simulink model "FODTfiiting"  (R2019a)
settings: Solver=ode2  StartTime=0.0  StopTime=300  FixedStep=0.1  RelTol=1e-3
settings Model: Creator=HP  LastModifiedBy=swastik
settings DataIOCC: ReturnWorkspaceOutputs=off
settings DebuggingCC: ArithmeticOperatorsInVariantConditions=warning

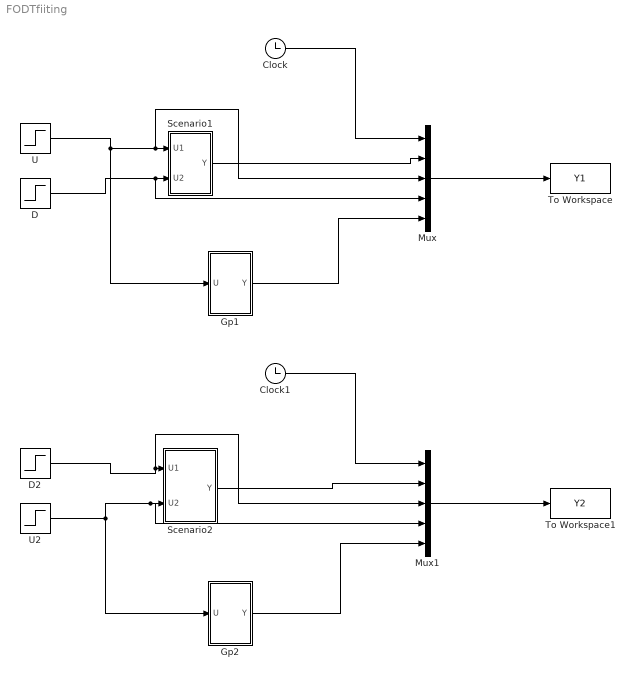
== system FODTfiiting ==
  Clock : Clock
  Clock1 : Clock
  D : Step  Time=0  After=0  SampleTime=0
  D2 : Step  Time=0  After=0  SampleTime=0
  Gp1 : Subsystem  mask{K=1.9886, T=17.4, D=14}
      mask prompts: K "Gain"; T "Lag Time"; D "Dead Time"
  Gp2 : Subsystem  mask{K2=0.9894, T2=26.1, D2=20.6}
      mask prompts: K2 "Gain"; T2 "Lag time"; D2 "Dead Time"
  Mux : Mux  Inputs=5
  Mux1 : Mux  Inputs=5
  Scenario1 : Subsystem
  Scenario2 : Subsystem
  To Workspace : ToWorkspace  VariableName=Y1  SampleTime=-1
  To Workspace1 : ToWorkspace  VariableName=Y2  SampleTime=-1
  U : Step  Time=0  SampleTime=0
  U2 : Step  Time=0  SampleTime=0
  wires:
  U/1 -> Gp1/1(U), Mux/3, Scenario1/1(U1)
  D/1 -> Mux/4, Scenario1/2(U2)
  Clock/1 -> Mux/1
  Scenario1/1(Y) -> Mux/2
  Mux/1 -> To Workspace/1
  Mux1/1 -> To Workspace1/1
  Scenario2/1(Y) -> Mux1/2
  D2/1 -> Mux1/3, Scenario2/1(U1)
  U2/1 -> Gp2/1(U), Mux1/4, Scenario2/2(U2)
  Clock1/1 -> Mux1/1
  Gp1/1(Y) -> Mux/5
  Gp2/1(Y) -> Mux1/5

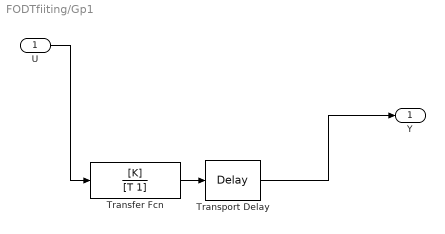
== system FODTfiiting/Gp1 ==
  U : Inport
  Transfer Fcn : TransferFcn  Numerator=[K]  Denominator=[T 1]
  Transport Delay : TransportDelay  DelayTime=D
  Y : Outport
  wires:
  Transfer Fcn/1 -> Transport Delay/1
  U/1 -> Transfer Fcn/1
  Transport Delay/1 -> Y/1

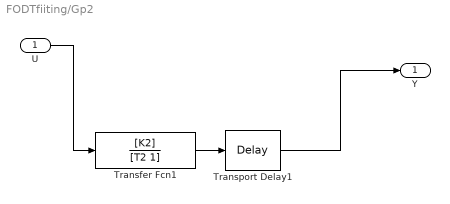
== system FODTfiiting/Gp2 ==
  U : Inport
  Transfer Fcn1 : TransferFcn  Numerator=[K2]  Denominator=[T2 1]
  Transport Delay1 : TransportDelay  DelayTime=D2
  Y : Outport
  wires:
  Transfer Fcn1/1 -> Transport Delay1/1
  Transport Delay1/1 -> Y/1
  U/1 -> Transfer Fcn1/1

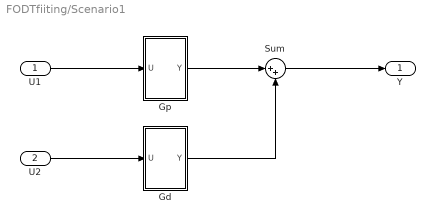
== system FODTfiiting/Scenario1 ==
  U1 : Inport
  U2 : Inport  Port=2
  Gd : Subsystem  mask{K1=0.45, K2=0.45, T1=0.3, T2=0.3, K=1/17e-4}
      mask prompts: K1 "Forward Gain"; K2 "Rev Gain"; T1 "Forward Time Constt"; T2 "Rev Time Constt"; K "Scaling Gain"
  Gp : Subsystem  mask{K1=0.45, K2=0.45, T1=0.2, T2=0.2, K=2.01/17e-4}
      mask prompts: K1 "Forward Gain"; K2 "Rev Gain"; T1 "Forward Time Constt"; T2 "Rev Time Constt"; K "Scaling Gain"
  Sum : Sum  Inputs=|++
  Y : Outport
  wires:
  Gd/1(Y) -> Sum/2
  Sum/1 -> Y/1
  Gp/1(Y) -> Sum/1
  U1/1 -> Gp/1(U)
  U2/1 -> Gd/1(U)

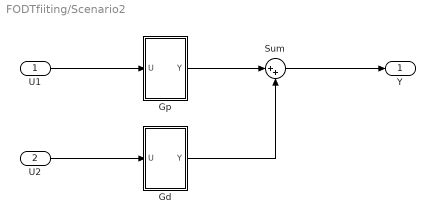
== system FODTfiiting/Scenario2 ==
  U1 : Inport
  U2 : Inport  Port=2
  Gd : Subsystem  mask{K1=0.45, K2=0.45, T1=0.3, T2=0.3, K=1/17e-4}
      mask prompts: K1 "Forward Gain"; K2 "Rev Gain"; T1 "Forward Time Constt"; T2 "Rev Time Constt"; K "Scaling Gain"
  Gp : Subsystem  mask{K1=0.45, K2=0.45, T1=0.2, T2=0.2, K=2.01/17e-4}
      mask prompts: K1 "Forward Gain"; K2 "Rev Gain"; T1 "Forward Time Constt"; T2 "Rev Time Constt"; K "Scaling Gain"
  Sum : Sum  Inputs=|++
  Y : Outport
  wires:
  Gd/1(Y) -> Sum/2
  Sum/1 -> Y/1
  Gp/1(Y) -> Sum/1
  U1/1 -> Gp/1(U)
  U2/1 -> Gd/1(U)

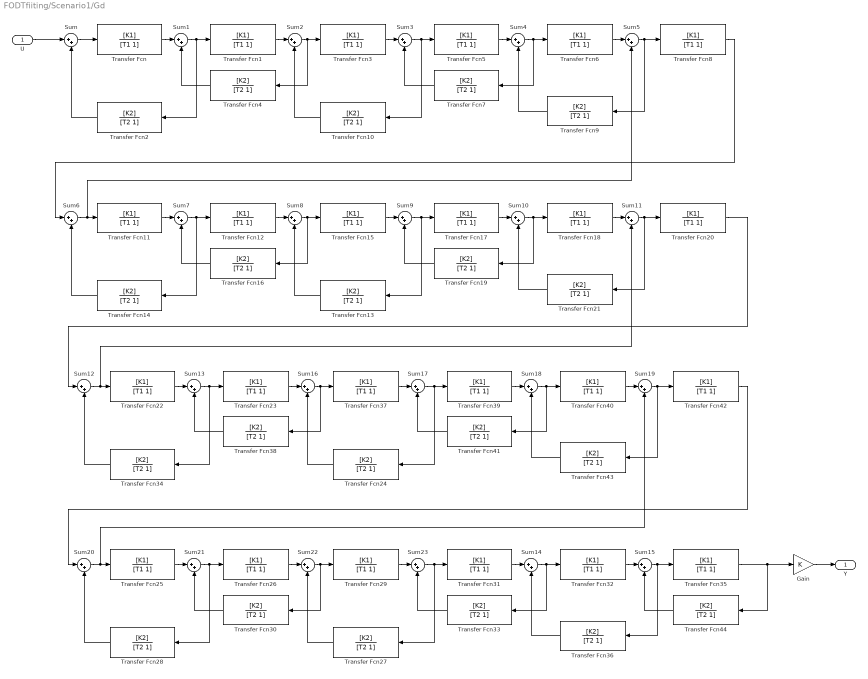
== system FODTfiiting/Scenario1/Gd ==
  U : Inport
  Gain : Gain  Gain=K
  Sum{,1..23} (24 alike) : Sum  Inputs=|++
  Transfer Fcn{,1,3,5..6,8,11..12,15,17..18,20,22..23,25..26,29,31..32,35,37,39..40,42} (24 alike) : TransferFcn  Numerator=[K1]  Denominator=[T1 1]
  Transfer Fcn{2,4,7,9..10,13..14,16,19,21,24,27..28,30,33..34,36,38,41,43..44} (21 alike) : TransferFcn  Numerator=[K2]  Denominator=[T2 1]
  Y : Outport
  wires:
  Transfer Fcn14/1 -> Sum6/2
  Transfer Fcn13/1 -> Sum8/2
  Transfer Fcn18/1 -> Sum11/1
  Transfer Fcn1/1 -> Sum2/1
  Sum18/1 -> Transfer Fcn41/1, Transfer Fcn40/1
  Sum21/1 -> Transfer Fcn28/1, Transfer Fcn26/1
  Transfer Fcn26/1 -> Sum22/1
  Transfer Fcn15/1 -> Sum9/1
  Sum13/1 -> Transfer Fcn34/1, Transfer Fcn23/1
  Sum7/1 -> Transfer Fcn14/1, Transfer Fcn12/1
  Sum8/1 -> Transfer Fcn16/1, Transfer Fcn15/1
  Transfer Fcn20/1 -> Sum12/1
  Sum20/1 -> Sum19/2, Transfer Fcn25/1
  Transfer Fcn9/1 -> Sum4/2
  Transfer Fcn25/1 -> Sum21/1
  Sum12/1 -> Sum11/2, Transfer Fcn22/1
  Transfer Fcn12/1 -> Sum8/1
  Transfer Fcn16/1 -> Sum7/2
  Transfer Fcn44/1 -> Sum15/2
  Transfer Fcn39/1 -> Sum18/1
  Sum2/1 -> Transfer Fcn4/1, Transfer Fcn3/1
  Transfer Fcn38/1 -> Sum13/2
  Sum17/1 -> Transfer Fcn24/1, Transfer Fcn39/1
  Sum9/1 -> Transfer Fcn13/1, Transfer Fcn17/1
  Transfer Fcn35/1 -> Gain/1, Transfer Fcn44/1
  Sum11/1 -> Transfer Fcn21/1, Transfer Fcn20/1
  Transfer Fcn42/1 -> Sum20/1
  Sum1/1 -> Transfer Fcn2/1, Transfer Fcn1/1
  Sum15/1 -> Transfer Fcn36/1, Transfer Fcn35/1
  Transfer Fcn27/1 -> Sum22/2
  Transfer Fcn24/1 -> Sum16/2
  Transfer Fcn31/1 -> Sum14/1
  Transfer Fcn23/1 -> Sum16/1
  Sum14/1 -> Transfer Fcn33/1, Transfer Fcn32/1
  Sum23/1 -> Transfer Fcn27/1, Transfer Fcn31/1
  Transfer Fcn40/1 -> Sum19/1
  Sum16/1 -> Transfer Fcn38/1, Transfer Fcn37/1
  Transfer Fcn22/1 -> Sum13/1
  Transfer Fcn34/1 -> Sum12/2
  Transfer Fcn37/1 -> Sum17/1
  Transfer Fcn33/1 -> Sum23/2
  Transfer Fcn41/1 -> Sum17/2
  Sum4/1 -> Transfer Fcn7/1, Transfer Fcn6/1
  Transfer Fcn36/1 -> Sum14/2
  Sum10/1 -> Transfer Fcn19/1, Transfer Fcn18/1
  Sum22/1 -> Transfer Fcn30/1, Transfer Fcn29/1
  Transfer Fcn6/1 -> Sum5/1
  Transfer Fcn29/1 -> Sum23/1
  Transfer Fcn2/1 -> Sum/2
  Transfer Fcn28/1 -> Sum20/2
  Transfer Fcn17/1 -> Sum10/1
  Transfer Fcn30/1 -> Sum21/2
  Transfer Fcn43/1 -> Sum18/2
  Transfer Fcn5/1 -> Sum4/1
  Sum19/1 -> Transfer Fcn43/1, Transfer Fcn42/1
  Sum3/1 -> Transfer Fcn10/1, Transfer Fcn5/1
  Transfer Fcn32/1 -> Sum15/1
  Sum6/1 -> Sum5/2, Transfer Fcn11/1
  Transfer Fcn/1 -> Sum1/1
  Transfer Fcn21/1 -> Sum10/2
  Sum5/1 -> Transfer Fcn9/1, Transfer Fcn8/1
  Transfer Fcn7/1 -> Sum3/2
  Transfer Fcn4/1 -> Sum1/2
  Transfer Fcn11/1 -> Sum7/1
  Transfer Fcn10/1 -> Sum2/2
  Transfer Fcn3/1 -> Sum3/1
  Transfer Fcn8/1 -> Sum6/1
  Transfer Fcn19/1 -> Sum9/2
  Sum/1 -> Transfer Fcn/1
  Gain/1 -> Y/1
  U/1 -> Sum/1

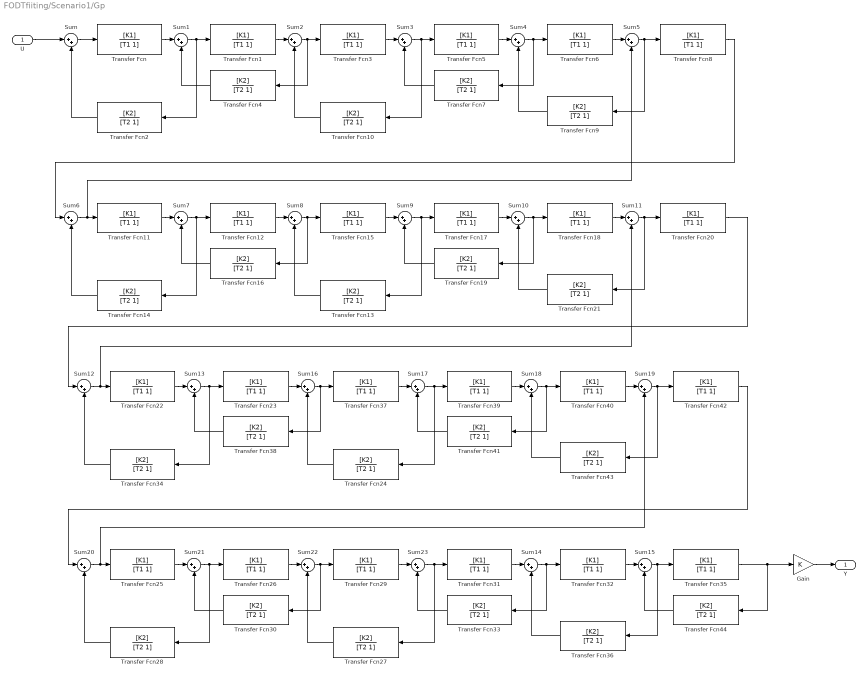
== system FODTfiiting/Scenario1/Gp ==
  U : Inport
  Gain : Gain  Gain=K
  Sum{,1..23} (24 alike) : Sum  Inputs=|++
  Transfer Fcn{,1,3,5..6,8,11..12,15,17..18,20,22..23,25..26,29,31..32,35,37,39..40,42} (24 alike) : TransferFcn  Numerator=[K1]  Denominator=[T1 1]
  Transfer Fcn{2,4,7,9..10,13..14,16,19,21,24,27..28,30,33..34,36,38,41,43..44} (21 alike) : TransferFcn  Numerator=[K2]  Denominator=[T2 1]
  Y : Outport
  wires:
  Transfer Fcn14/1 -> Sum6/2
  Transfer Fcn13/1 -> Sum8/2
  Transfer Fcn18/1 -> Sum11/1
  Transfer Fcn1/1 -> Sum2/1
  Sum18/1 -> Transfer Fcn41/1, Transfer Fcn40/1
  Sum21/1 -> Transfer Fcn28/1, Transfer Fcn26/1
  Transfer Fcn26/1 -> Sum22/1
  Transfer Fcn15/1 -> Sum9/1
  Sum13/1 -> Transfer Fcn34/1, Transfer Fcn23/1
  Sum7/1 -> Transfer Fcn14/1, Transfer Fcn12/1
  Sum8/1 -> Transfer Fcn16/1, Transfer Fcn15/1
  Transfer Fcn20/1 -> Sum12/1
  Sum20/1 -> Sum19/2, Transfer Fcn25/1
  Transfer Fcn9/1 -> Sum4/2
  Transfer Fcn25/1 -> Sum21/1
  Sum12/1 -> Sum11/2, Transfer Fcn22/1
  Transfer Fcn12/1 -> Sum8/1
  Transfer Fcn16/1 -> Sum7/2
  Transfer Fcn44/1 -> Sum15/2
  Transfer Fcn39/1 -> Sum18/1
  Sum2/1 -> Transfer Fcn4/1, Transfer Fcn3/1
  Transfer Fcn38/1 -> Sum13/2
  Sum17/1 -> Transfer Fcn24/1, Transfer Fcn39/1
  Sum9/1 -> Transfer Fcn13/1, Transfer Fcn17/1
  Transfer Fcn35/1 -> Gain/1, Transfer Fcn44/1
  Sum11/1 -> Transfer Fcn21/1, Transfer Fcn20/1
  Transfer Fcn42/1 -> Sum20/1
  Sum1/1 -> Transfer Fcn2/1, Transfer Fcn1/1
  Sum15/1 -> Transfer Fcn36/1, Transfer Fcn35/1
  Transfer Fcn27/1 -> Sum22/2
  Transfer Fcn24/1 -> Sum16/2
  Transfer Fcn31/1 -> Sum14/1
  Transfer Fcn23/1 -> Sum16/1
  Sum14/1 -> Transfer Fcn33/1, Transfer Fcn32/1
  Sum23/1 -> Transfer Fcn27/1, Transfer Fcn31/1
  Transfer Fcn40/1 -> Sum19/1
  Sum16/1 -> Transfer Fcn38/1, Transfer Fcn37/1
  Transfer Fcn22/1 -> Sum13/1
  Transfer Fcn34/1 -> Sum12/2
  Transfer Fcn37/1 -> Sum17/1
  Transfer Fcn33/1 -> Sum23/2
  Transfer Fcn41/1 -> Sum17/2
  Sum4/1 -> Transfer Fcn7/1, Transfer Fcn6/1
  Transfer Fcn36/1 -> Sum14/2
  Sum10/1 -> Transfer Fcn19/1, Transfer Fcn18/1
  Sum22/1 -> Transfer Fcn30/1, Transfer Fcn29/1
  Transfer Fcn6/1 -> Sum5/1
  Transfer Fcn29/1 -> Sum23/1
  Transfer Fcn2/1 -> Sum/2
  Transfer Fcn28/1 -> Sum20/2
  Transfer Fcn17/1 -> Sum10/1
  Transfer Fcn30/1 -> Sum21/2
  Transfer Fcn43/1 -> Sum18/2
  Transfer Fcn5/1 -> Sum4/1
  Sum19/1 -> Transfer Fcn43/1, Transfer Fcn42/1
  Sum3/1 -> Transfer Fcn10/1, Transfer Fcn5/1
  Transfer Fcn32/1 -> Sum15/1
  Sum6/1 -> Sum5/2, Transfer Fcn11/1
  Transfer Fcn/1 -> Sum1/1
  Transfer Fcn21/1 -> Sum10/2
  Sum5/1 -> Transfer Fcn9/1, Transfer Fcn8/1
  Transfer Fcn7/1 -> Sum3/2
  Transfer Fcn4/1 -> Sum1/2
  Transfer Fcn11/1 -> Sum7/1
  Transfer Fcn10/1 -> Sum2/2
  Transfer Fcn3/1 -> Sum3/1
  Transfer Fcn8/1 -> Sum6/1
  Transfer Fcn19/1 -> Sum9/2
  Sum/1 -> Transfer Fcn/1
  Gain/1 -> Y/1
  U/1 -> Sum/1

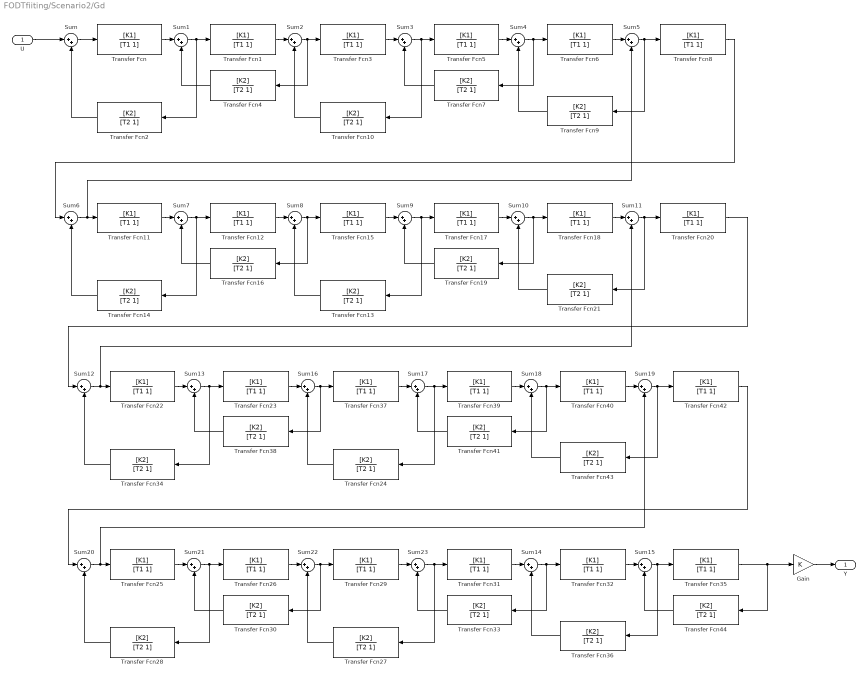
== system FODTfiiting/Scenario2/Gd ==
  U : Inport
  Gain : Gain  Gain=K
  Sum{,1..23} (24 alike) : Sum  Inputs=|++
  Transfer Fcn{,1,3,5..6,8,11..12,15,17..18,20,22..23,25..26,29,31..32,35,37,39..40,42} (24 alike) : TransferFcn  Numerator=[K1]  Denominator=[T1 1]
  Transfer Fcn{2,4,7,9..10,13..14,16,19,21,24,27..28,30,33..34,36,38,41,43..44} (21 alike) : TransferFcn  Numerator=[K2]  Denominator=[T2 1]
  Y : Outport
  wires:
  Transfer Fcn14/1 -> Sum6/2
  Transfer Fcn13/1 -> Sum8/2
  Transfer Fcn18/1 -> Sum11/1
  Transfer Fcn1/1 -> Sum2/1
  Sum18/1 -> Transfer Fcn41/1, Transfer Fcn40/1
  Sum21/1 -> Transfer Fcn28/1, Transfer Fcn26/1
  Transfer Fcn26/1 -> Sum22/1
  Transfer Fcn15/1 -> Sum9/1
  Sum13/1 -> Transfer Fcn34/1, Transfer Fcn23/1
  Sum7/1 -> Transfer Fcn14/1, Transfer Fcn12/1
  Sum8/1 -> Transfer Fcn16/1, Transfer Fcn15/1
  Transfer Fcn20/1 -> Sum12/1
  Sum20/1 -> Sum19/2, Transfer Fcn25/1
  Transfer Fcn9/1 -> Sum4/2
  Transfer Fcn25/1 -> Sum21/1
  Sum12/1 -> Sum11/2, Transfer Fcn22/1
  Transfer Fcn12/1 -> Sum8/1
  Transfer Fcn16/1 -> Sum7/2
  Transfer Fcn44/1 -> Sum15/2
  Transfer Fcn39/1 -> Sum18/1
  Sum2/1 -> Transfer Fcn4/1, Transfer Fcn3/1
  Transfer Fcn38/1 -> Sum13/2
  Sum17/1 -> Transfer Fcn24/1, Transfer Fcn39/1
  Sum9/1 -> Transfer Fcn13/1, Transfer Fcn17/1
  Transfer Fcn35/1 -> Gain/1, Transfer Fcn44/1
  Sum11/1 -> Transfer Fcn21/1, Transfer Fcn20/1
  Transfer Fcn42/1 -> Sum20/1
  Sum1/1 -> Transfer Fcn2/1, Transfer Fcn1/1
  Sum15/1 -> Transfer Fcn36/1, Transfer Fcn35/1
  Transfer Fcn27/1 -> Sum22/2
  Transfer Fcn24/1 -> Sum16/2
  Transfer Fcn31/1 -> Sum14/1
  Transfer Fcn23/1 -> Sum16/1
  Sum14/1 -> Transfer Fcn33/1, Transfer Fcn32/1
  Sum23/1 -> Transfer Fcn27/1, Transfer Fcn31/1
  Transfer Fcn40/1 -> Sum19/1
  Sum16/1 -> Transfer Fcn38/1, Transfer Fcn37/1
  Transfer Fcn22/1 -> Sum13/1
  Transfer Fcn34/1 -> Sum12/2
  Transfer Fcn37/1 -> Sum17/1
  Transfer Fcn33/1 -> Sum23/2
  Transfer Fcn41/1 -> Sum17/2
  Sum4/1 -> Transfer Fcn7/1, Transfer Fcn6/1
  Transfer Fcn36/1 -> Sum14/2
  Sum10/1 -> Transfer Fcn19/1, Transfer Fcn18/1
  Sum22/1 -> Transfer Fcn30/1, Transfer Fcn29/1
  Transfer Fcn6/1 -> Sum5/1
  Transfer Fcn29/1 -> Sum23/1
  Transfer Fcn2/1 -> Sum/2
  Transfer Fcn28/1 -> Sum20/2
  Transfer Fcn17/1 -> Sum10/1
  Transfer Fcn30/1 -> Sum21/2
  Transfer Fcn43/1 -> Sum18/2
  Transfer Fcn5/1 -> Sum4/1
  Sum19/1 -> Transfer Fcn43/1, Transfer Fcn42/1
  Sum3/1 -> Transfer Fcn10/1, Transfer Fcn5/1
  Transfer Fcn32/1 -> Sum15/1
  Sum6/1 -> Sum5/2, Transfer Fcn11/1
  Transfer Fcn/1 -> Sum1/1
  Transfer Fcn21/1 -> Sum10/2
  Sum5/1 -> Transfer Fcn9/1, Transfer Fcn8/1
  Transfer Fcn7/1 -> Sum3/2
  Transfer Fcn4/1 -> Sum1/2
  Transfer Fcn11/1 -> Sum7/1
  Transfer Fcn10/1 -> Sum2/2
  Transfer Fcn3/1 -> Sum3/1
  Transfer Fcn8/1 -> Sum6/1
  Transfer Fcn19/1 -> Sum9/2
  Sum/1 -> Transfer Fcn/1
  Gain/1 -> Y/1
  U/1 -> Sum/1

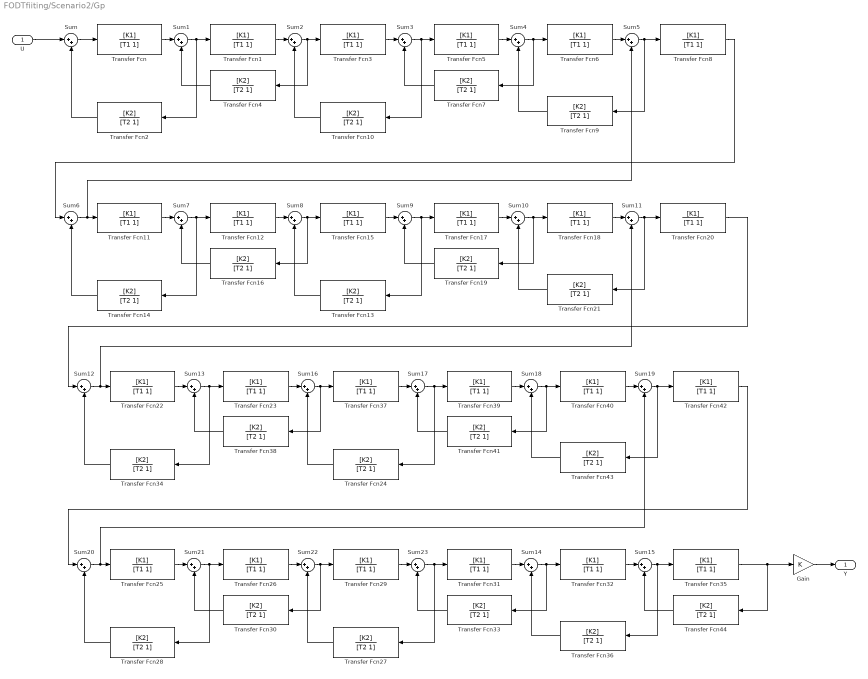
== system FODTfiiting/Scenario2/Gp ==
  U : Inport
  Gain : Gain  Gain=K
  Sum{,1..23} (24 alike) : Sum  Inputs=|++
  Transfer Fcn{,1,3,5..6,8,11..12,15,17..18,20,22..23,25..26,29,31..32,35,37,39..40,42} (24 alike) : TransferFcn  Numerator=[K1]  Denominator=[T1 1]
  Transfer Fcn{2,4,7,9..10,13..14,16,19,21,24,27..28,30,33..34,36,38,41,43..44} (21 alike) : TransferFcn  Numerator=[K2]  Denominator=[T2 1]
  Y : Outport
  wires:
  Transfer Fcn14/1 -> Sum6/2
  Transfer Fcn13/1 -> Sum8/2
  Transfer Fcn18/1 -> Sum11/1
  Transfer Fcn1/1 -> Sum2/1
  Sum18/1 -> Transfer Fcn41/1, Transfer Fcn40/1
  Sum21/1 -> Transfer Fcn28/1, Transfer Fcn26/1
  Transfer Fcn26/1 -> Sum22/1
  Transfer Fcn15/1 -> Sum9/1
  Sum13/1 -> Transfer Fcn34/1, Transfer Fcn23/1
  Sum7/1 -> Transfer Fcn14/1, Transfer Fcn12/1
  Sum8/1 -> Transfer Fcn16/1, Transfer Fcn15/1
  Transfer Fcn20/1 -> Sum12/1
  Sum20/1 -> Sum19/2, Transfer Fcn25/1
  Transfer Fcn9/1 -> Sum4/2
  Transfer Fcn25/1 -> Sum21/1
  Sum12/1 -> Sum11/2, Transfer Fcn22/1
  Transfer Fcn12/1 -> Sum8/1
  Transfer Fcn16/1 -> Sum7/2
  Transfer Fcn44/1 -> Sum15/2
  Transfer Fcn39/1 -> Sum18/1
  Sum2/1 -> Transfer Fcn4/1, Transfer Fcn3/1
  Transfer Fcn38/1 -> Sum13/2
  Sum17/1 -> Transfer Fcn24/1, Transfer Fcn39/1
  Sum9/1 -> Transfer Fcn13/1, Transfer Fcn17/1
  Transfer Fcn35/1 -> Gain/1, Transfer Fcn44/1
  Sum11/1 -> Transfer Fcn21/1, Transfer Fcn20/1
  Transfer Fcn42/1 -> Sum20/1
  Sum1/1 -> Transfer Fcn2/1, Transfer Fcn1/1
  Sum15/1 -> Transfer Fcn36/1, Transfer Fcn35/1
  Transfer Fcn27/1 -> Sum22/2
  Transfer Fcn24/1 -> Sum16/2
  Transfer Fcn31/1 -> Sum14/1
  Transfer Fcn23/1 -> Sum16/1
  Sum14/1 -> Transfer Fcn33/1, Transfer Fcn32/1
  Sum23/1 -> Transfer Fcn27/1, Transfer Fcn31/1
  Transfer Fcn40/1 -> Sum19/1
  Sum16/1 -> Transfer Fcn38/1, Transfer Fcn37/1
  Transfer Fcn22/1 -> Sum13/1
  Transfer Fcn34/1 -> Sum12/2
  Transfer Fcn37/1 -> Sum17/1
  Transfer Fcn33/1 -> Sum23/2
  Transfer Fcn41/1 -> Sum17/2
  Sum4/1 -> Transfer Fcn7/1, Transfer Fcn6/1
  Transfer Fcn36/1 -> Sum14/2
  Sum10/1 -> Transfer Fcn19/1, Transfer Fcn18/1
  Sum22/1 -> Transfer Fcn30/1, Transfer Fcn29/1
  Transfer Fcn6/1 -> Sum5/1
  Transfer Fcn29/1 -> Sum23/1
  Transfer Fcn2/1 -> Sum/2
  Transfer Fcn28/1 -> Sum20/2
  Transfer Fcn17/1 -> Sum10/1
  Transfer Fcn30/1 -> Sum21/2
  Transfer Fcn43/1 -> Sum18/2
  Transfer Fcn5/1 -> Sum4/1
  Sum19/1 -> Transfer Fcn43/1, Transfer Fcn42/1
  Sum3/1 -> Transfer Fcn10/1, Transfer Fcn5/1
  Transfer Fcn32/1 -> Sum15/1
  Sum6/1 -> Sum5/2, Transfer Fcn11/1
  Transfer Fcn/1 -> Sum1/1
  Transfer Fcn21/1 -> Sum10/2
  Sum5/1 -> Transfer Fcn9/1, Transfer Fcn8/1
  Transfer Fcn7/1 -> Sum3/2
  Transfer Fcn4/1 -> Sum1/2
  Transfer Fcn11/1 -> Sum7/1
  Transfer Fcn10/1 -> Sum2/2
  Transfer Fcn3/1 -> Sum3/1
  Transfer Fcn8/1 -> Sum6/1
  Transfer Fcn19/1 -> Sum9/2
  Sum/1 -> Transfer Fcn/1
  Gain/1 -> Y/1
  U/1 -> Sum/1
